simulink model "simulation4coders"  (R2022b)
settings: Solver=VariableStepAuto  StartTime=0.0  StopTime=10.0  RelTol=1e-3
libraries: simulink x1
settings Model: Creator=LeonK  LastModifiedBy=LeonK

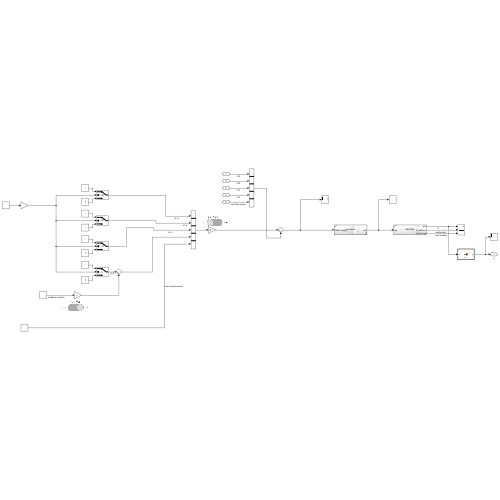
[thumbnail: Simulink's stored preview of the top-level diagram]
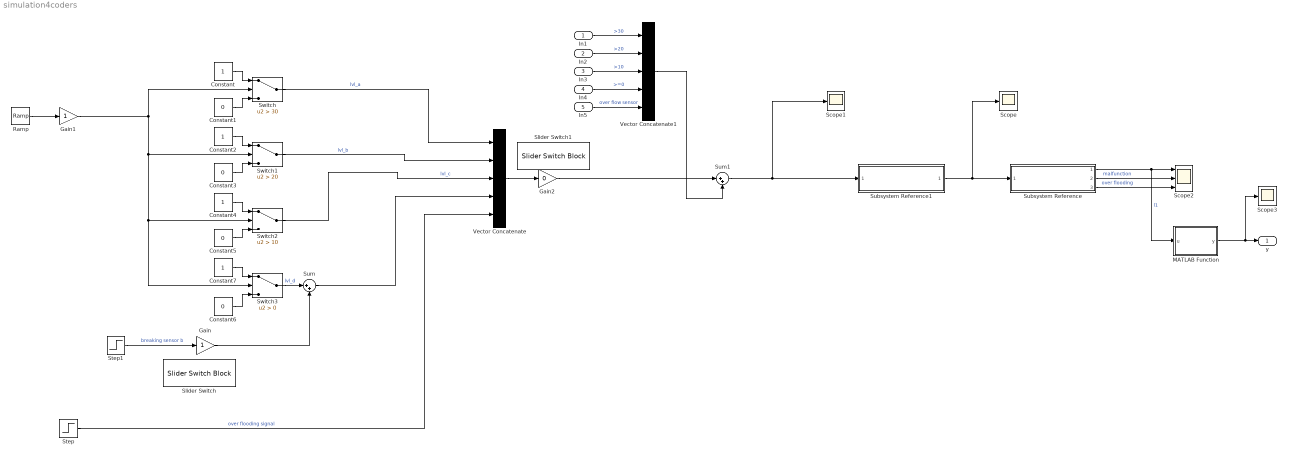
== system simulation4coders ==
  In1 : Inport
  In2 : Inport  Port=2
  In3 : Inport  Port=3
  In4 : Inport  Port=4
  In5 : Inport  Port=5
  Constant{,2,4,7} (4 alike) : Constant
  Constant{1,3,5..6} (4 alike) : Constant  Value=0
  Gain : Gain
  Gain1 : Gain
  Gain2 : Gain  Gain=0
  MATLAB Function : MATLAB Function  TreatAsAtomicUnit=on
  Ramp : simulink/Sources/Ramp  slope=5  start=0  InitialOutput=0
  Scope : Scope
  Scope1 : Scope
  Scope2 : Scope  NumInputPorts=3
  Scope3 : Scope
  Slider Switch : SliderSwitchBlock
      settings: Values={{'Off', 'On'}, [0 1]}
  Slider Switch1 : SliderSwitchBlock
      settings: Values={{'Off', 'On'}, [0 1]}
  Step : Step  Time=10  SampleTime=0
  Step1 : Step  Time=7  After=-1  SampleTime=0
  Subsystem Reference : Subsystem  ReferencedSubsystem=decoder
  Subsystem Reference1 : Subsystem  ReferencedSubsystem=encoder
  Sum : Sum  Inputs=|++
  Sum1 : Sum  Inputs=|++
  Switch : Switch  Criteria=u2 > Threshold  Threshold=30  SaturateOnIntegerOverflow=off  InputSameDT=off
  Switch1 : Switch  Criteria=u2 > Threshold  Threshold=20  SaturateOnIntegerOverflow=off  InputSameDT=off
  Switch2 : Switch  Criteria=u2 > Threshold  Threshold=10  SaturateOnIntegerOverflow=off  InputSameDT=off
  Switch3 : Switch  Criteria=u2 > Threshold  SaturateOnIntegerOverflow=off  InputSameDT=off
  Vector Concatenate : Concatenate  NumInputs=5
  Vector Concatenate1 : Concatenate  NumInputs=5
  y : Outport
  wires:
  Subsystem Reference1/1 -> Scope/1, Subsystem Reference/1
  Constant/1 -> Switch/1
  Constant1/1 -> Switch/3
  Constant2/1 -> Switch1/1
  Constant3/1 -> Switch1/3
  Constant4/1 -> Switch2/1
  Constant5/1 -> Switch2/3
  Constant7/1 -> Switch3/1
  Constant6/1 -> Switch3/3
  Switch/1 -> Vector Concatenate/1  "lvl_a"
  Switch2/1 -> Vector Concatenate/3  "lvl_c"
  Vector Concatenate/1 -> Gain2/1
  Ramp/1 -> Gain1/1
  Subsystem Reference/1 -> MATLAB Function/1(u), Scope2/1  "l1"
  Step/1 -> Vector Concatenate/5  "over flooding signal"
  Subsystem Reference/2 -> Scope2/2  "malfunction"
  Subsystem Reference/3 -> Scope2/3  "over flooding"
  Switch1/1 -> Vector Concatenate/2  "lvl_b"
  Switch3/1 -> Sum/1  "lvl_d"
  Sum/1 -> Vector Concatenate/4
  Step1/1 -> Gain/1  "breaking sensor b"
  MATLAB Function/1(y) -> Scope3/1, y/1
  Gain/1 -> Sum/2
  Gain1/1 -> Switch2/2, Switch3/2, Switch1/2, Switch/2
  Gain2/1 -> Sum1/1
  Sum1/1 -> Scope1/1, Subsystem Reference1/1
  Vector Concatenate1/1 -> Sum1/2
  In1/1 -> Vector Concatenate1/1  ">30"
  In2/1 -> Vector Concatenate1/2  ">20"
  In3/1 -> Vector Concatenate1/3  ">10"
  In4/1 -> Vector Concatenate1/4  ">=0"
  In5/1 -> Vector Concatenate1/5  "over flow sensor"

== matlab function simulation4coders/MATLAB Function ==
  data: u input; y output
function y = fcn(u)
    if (u==3)
        y = 5;
    elseif (u==4 || u==5)
        y = 10;
    else
        y = 0;
    end
